simulink library "test_function"  (R2016b)
settings: Solver=VariableStepAuto  StartTime=0.0  StopTime=10.0  RelTol=1e-3
settings Model: Creator=Jacob  LastModifiedBy=Jacob

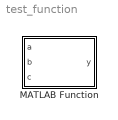
== system test_function ==
  MATLAB Function : MATLAB Function  TreatAsAtomicUnit=on

== matlab function test_function/MATLAB Function ==
  data: a input; y output; b input; c input
function y = fcn(a,b,c)
a = a;
b = b;
c = c;

u = a + b+c;
y = u;
